simulink model "Blinker_31_exp_start"  (R2020b)
settings: Solver=FixedStepDiscrete  StartTime=0.0  StopTime=10.0  FixedStep=Ts  RelTol=1e-3  EnableMultiTasking=on
PreLoadFcn:
  | Ts = 0.05;
  | Ts_1 = 0.05;   % for runnable blink_signal
  | Ts_2 = 1;       % for runnable validate_ignition
  | 
  | SetEnumTypeBlink;
undefined symbols (not defined in the file or in its folder): BlinkerValues
libraries: simulink x1
settings Model: SimSIMDOptimization=Portable  Creator=urempel  LastModifiedBy=bnewman
settings DataIOCC: LimitDataPoints=on  SaveFormat=Array  ReturnWorkspaceOutputs=off
settings OptimizationCC: LifeSpan=1  EfficientTunableParamExpr=on
settings DebuggingCC: SolverPrmCheckMsg=warning  AllowSymbolicDim=off  SFUnexpectedBacktrackingDiag=warning  SFNoUnconditionalDefaultTransitionDiag=warning  SFExecutionAtInitializationDiag=none  ArithmeticOperatorsInVariantConditions=warning
settings ModelReferenceCC: PropagateSignalLabelsOutOfModel=off
settings SFSimCC: SimUseLocalCustomCode=off  SimGenImportedTypeDefs=on  MATLABDynamicMemAlloc=off  CustomCodeUndefinedFunction=UseInterfaceOnly
settings RTWCC: Description=Embedded Coder  SystemTargetFile=ert.tlc  GenCodeOnly=on  TemplateMakefile=ert_default_tmf  RTWUseLocalCustomCode=off  IncludeHyperlinkInReport=on
settings CodeAppCC: IgnoreCustomStorageClasses=off  StateflowObjectComments=on
settings ERTTargetCC: MultiwordLength=2048  GenerateSampleERTMain=on  ERTCustomFileTemplate=example_file_process.tlc  ConvertIfToSwitch=off  SuppressUnreachableDefaultCases=off
settings ConfigComp: CovMetricSettings=dw  CovSaveCumulativeToWorkspaceVar=on  CovSaveSingleToWorkspaceVar=on  CovExternalEMLEnable=off  CovSFcnEnable=off

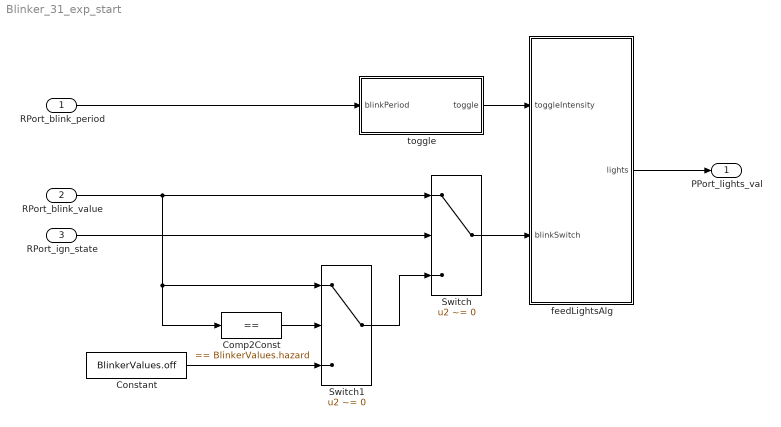
== system Blinker_31_exp_start ==
  RPort_blink_period : Inport  OutDataTypeStr=uint32
      settings: AttributesFormatString=%<OutDataTypeStr>
  RPort_blink_value : Inport  Port=2  OutDataTypeStr=Enum: BlinkerValues
      settings: AttributesFormatString=%<OutDataTypeStr>
  RPort_ign_state : Inport  Port=3  OutDataTypeStr=boolean
      settings: AttributesFormatString=%<OutDataTypeStr>
  Comp2Const : simulink/Logic and Bit Operations/Compare To Constant  relop===  const=BlinkerValues.hazard  OutDataTypeStr=boolean
  Constant : Constant  Value=BlinkerValues.off
      settings: AttributesFormatString=%<OutDataTypeStr>
  Switch : Switch  Criteria=u2 ~= 0
  Switch1 : Switch  Criteria=u2 ~= 0
  feedLightsAlg : MATLAB Function  TreatAsAtomicUnit=on
  toggle : Stateflow chart  TreatAsAtomicUnit=on
  PPort_lights_val : Outport  InitialOutput=0
  wires:
  feedLightsAlg/1(lights) -> PPort_lights_val/1
  RPort_blink_value/1 -> Switch1/1, Comp2Const/1, Switch/1
  Comp2Const/1 -> Switch1/2
  Constant/1 -> Switch1/3
  RPort_ign_state/1 -> Switch/2
  Switch/1 -> feedLightsAlg/2(blinkSwitch)
  toggle/1(toggle) -> feedLightsAlg/1(toggleIntensity)
  RPort_blink_period/1 -> toggle/1(blinkPeriod)
  Switch1/1 -> Switch/3

== matlab function Blinker_31_exp_start/feedLightsAlg ==
  data: toggleIntensity input boolean; blinkSwitch input Enum: BlinkerValues; lights output boolean size=[1,2]
function lights = feedLightsAlg(toggleIntensity, blinkSwitch )
%#codegen
switch blinkSwitch
	case BlinkerValues.right
		lights = [false, toggleIntensity];
	case BlinkerValues.left
		lights = [toggleIntensity, false];
	case BlinkerValues.hazard
		lights = [toggleIntensity, toggleIntensity];
	otherwise
		lights = [false, false];
end

== stateflow chart Blinker_31_exp_start/toggle ==
  (default) -> (junction 2)
  (junction 2) -> (junction 7) [order 1] : [blinkPeriod <= cntr]
  (junction 2) -> (junction 3) [order 2] : {
      | cntr++;
      | }
  (junction 7) -> (junction 8) : {
      | toggle = !toggle;
      | cntr = 1;
      | }
  (junction 8) -> (junction 3)
  data: toggle output boolean =0; blinkPeriod input uint32; cntr local uint32 =0
